simulink library "PECommon"  (Simulink 7.6)
settings: Solver=ode45  StartTime=0.0  StopTime=10.0  RelTol=1e-3
undefined symbols (not defined in the file or in its folder): DiscIntNeverNeededParam, Hydride, Metal, Nickel, Ts, Ts_Discrete
libraries: powerlib x24, simulink x14, PECommon x7, powerlib_extras x7, electricdrivelib x1, simulink_extras x1
(part 2 of 2)

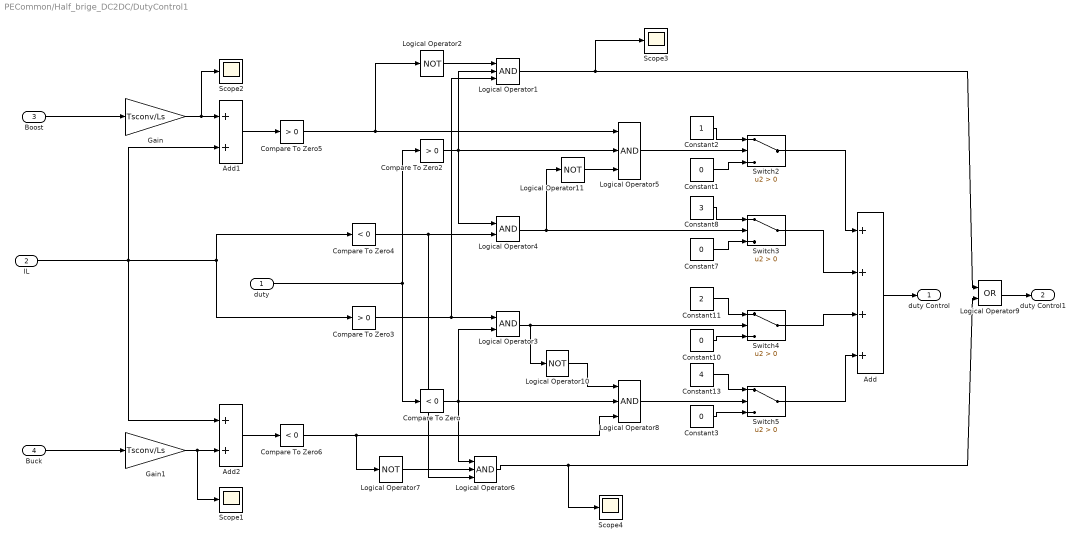
== system PECommon/Half_brige_DC2DC/DutyControl1 ==
  duty : Inport
  IL : Inport  Port=2
  Boost : Inport  Port=3
  Buck : Inport  Port=4
  Add : Sum  Inputs=++++
  Add1 : Sum
  Add2 : Sum
  Compare To Zero : simulink/Logic and Bit Operations/Compare To Zero  SystemSampleTime=-1  relop=<  LogicOutDataTypeMode=boolean  ZeroCross=off
  Compare To Zero2 : simulink/Logic and Bit Operations/Compare To Zero  SystemSampleTime=-1  relop=>  LogicOutDataTypeMode=boolean  ZeroCross=off
  Compare To Zero3 : simulink/Logic and Bit Operations/Compare To Zero  SystemSampleTime=-1  relop=>  LogicOutDataTypeMode=boolean  ZeroCross=off
  Compare To Zero4 : simulink/Logic and Bit Operations/Compare To Zero  SystemSampleTime=-1  relop=<  LogicOutDataTypeMode=boolean  ZeroCross=off
  Compare To Zero5 : simulink/Logic and Bit Operations/Compare To Zero  SystemSampleTime=-1  relop=>  LogicOutDataTypeMode=boolean  ZeroCross=off
  Compare To Zero6 : simulink/Logic and Bit Operations/Compare To Zero  SystemSampleTime=-1  relop=<  LogicOutDataTypeMode=boolean  ZeroCross=off
  Constant{1,3,7,10} (4 alike) : Constant  Value=0
  Constant11 : Constant  Value=2
  Constant13 : Constant  Value=4
  Constant2 : Constant
  Constant8 : Constant  Value=3
  Gain : Gain  Gain=Tsconv/Ls
  Gain1 : Gain  Gain=Tsconv/Ls
  Logical Operator{1,5..6,8} (4 alike) : Logic  Inputs=3  AllPortsSameDT=off  OutDataTypeStr=boolean
  Logical Operator{2,7,10..11} (4 alike) : Logic  Operator=NOT  AllPortsSameDT=off  OutDataTypeStr=boolean
  Logical Operator3 : Logic  AllPortsSameDT=off  OutDataTypeStr=boolean
  Logical Operator4 : Logic  AllPortsSameDT=off  OutDataTypeStr=boolean
  Logical Operator9 : Logic  Operator=OR  AllPortsSameDT=off  OutDataTypeStr=boolean
  Scope{1..4} (4 alike) : Scope
      Scope1 settings: SaveName=ScopeData15
      Scope2 settings: SaveName=ScopeData16
      Scope3 settings: SaveName=ScopeData17
      Scope4 settings: SaveName=ScopeData18
  Switch{2..5} (4 alike) : Switch  Criteria=u2 > Threshold  ZeroCross=off
  duty Control : Outport
  duty Control1 : Outport  Port=2
  wires:
  Constant7/1 -> Switch3/3
  Constant10/1 -> Switch4/3
  Constant11/1 -> Switch4/1
  Constant8/1 -> Switch3/1
  duty/1 -> Compare To Zero/1, Compare To Zero2/1
  Add/1 -> duty Control/1
  Constant1/1 -> Switch2/3
  Constant2/1 -> Switch2/1
  Constant3/1 -> Switch5/3
  Constant13/1 -> Switch5/1
  Compare To Zero/1 -> Logical Operator3/2, Logical Operator8/2, Logical Operator6/1
  Boost/1 -> Gain/1
  Gain/1 -> Add1/1, Scope2/1
  IL/1 -> Add1/2, Add2/1, Compare To Zero4/1, Compare To Zero3/1
  Logical Operator3/1 -> Logical Operator10/1, Switch4/2
  Compare To Zero3/1 -> Logical Operator1/3, Logical Operator3/1
  Compare To Zero2/1 -> Logical Operator4/1, Logical Operator5/2, Logical Operator1/2
  Logical Operator4/1 -> Switch3/2, Logical Operator11/1
  Compare To Zero4/1 -> Logical Operator6/3, Logical Operator4/2
  Add1/1 -> Compare To Zero5/1
  Logical Operator5/1 -> Switch2/2
  Switch3/1 -> Add/2
  Switch2/1 -> Add/1
  Buck/1 -> Gain1/1
  Add2/1 -> Compare To Zero6/1
  Gain1/1 -> Add2/2, Scope1/1
  Logical Operator8/1 -> Switch5/2
  Logical Operator10/1 -> Logical Operator8/1
  Logical Operator11/1 -> Logical Operator5/3
  Switch4/1 -> Add/3
  Switch5/1 -> Add/4
  Compare To Zero6/1 -> Logical Operator8/3, Logical Operator7/1
  Compare To Zero5/1 -> Logical Operator5/1, Logical Operator2/1
  Logical Operator2/1 -> Logical Operator1/1
  Logical Operator1/1 -> Scope3/1, Logical Operator9/1
  Logical Operator7/1 -> Logical Operator6/2
  Logical Operator6/1 -> Scope4/1, Logical Operator9/2
  Logical Operator9/1 -> duty Control1/1

== system PECommon/VSI2CSI/Value ==
  In1 : Inport
  Constant : Constant  Value=0
  Constant1 : Constant  Value=Value
  Switch : Switch  Criteria=u2 > Threshold
  Out1 : Outport
  wires:
  Switch/1 -> Out1/1
  In1/1 -> Switch/2
  Constant/1 -> Switch/3
  Constant1/1 -> Switch/1

== system PECommon/VSI2CSI/Value1 ==
  In1 : Inport
  Constant : Constant  Value=0
  Constant1 : Constant  Value=Value
  Switch : Switch  Criteria=u2 > Threshold
  Out1 : Outport
  wires:
  Constant1/1 -> Switch/1
  Constant/1 -> Switch/3
  In1/1 -> Switch/2
  Switch/1 -> Out1/1

== system PECommon/VSI2CSI/Value2 ==
  In1 : Inport
  Constant : Constant  Value=0
  Constant1 : Constant  Value=Value
  Switch : Switch  Criteria=u2 > Threshold
  Out1 : Outport
  wires:
  Switch/1 -> Out1/1
  In1/1 -> Switch/2
  Constant/1 -> Switch/3
  Constant1/1 -> Switch/1

== system PECommon/VSI2CSI/Value3 ==
  In1 : Inport
  Constant : Constant  Value=0
  Constant1 : Constant  Value=Value
  Switch : Switch  Criteria=u2 > Threshold
  Out1 : Outport
  wires:
  Constant1/1 -> Switch/1
  Constant/1 -> Switch/3
  In1/1 -> Switch/2
  Switch/1 -> Out1/1

== system PECommon/VSI2CSI/Value4 ==
  In1 : Inport
  Constant : Constant  Value=0
  Constant1 : Constant  Value=Value
  Switch : Switch  Criteria=u2 > Threshold
  Out1 : Outport
  wires:
  Switch/1 -> Out1/1
  In1/1 -> Switch/2
  Constant/1 -> Switch/3
  Constant1/1 -> Switch/1

== system PECommon/VSI2CSI/Value5 ==
  In1 : Inport
  Constant : Constant  Value=0
  Constant1 : Constant  Value=Value
  Switch : Switch  Criteria=u2 > Threshold
  Out1 : Outport
  wires:
  Constant1/1 -> Switch/1
  Constant/1 -> Switch/3
  In1/1 -> Switch/2
  Switch/1 -> Out1/1

== system PECommon/VSI2CSI/Value6 ==
  In1 : Inport
  Constant : Constant  Value=0
  Constant1 : Constant  Value=Value
  Switch : Switch  Criteria=u2 > Threshold
  Out1 : Outport
  wires:
  Constant1/1 -> Switch/1
  Constant/1 -> Switch/3
  In1/1 -> Switch/2
  Switch/1 -> Out1/1

== system PECommon/VSI2CSI/Value7 ==
  In1 : Inport
  Constant : Constant  Value=0
  Constant1 : Constant  Value=Value
  Switch : Switch  Criteria=u2 > Threshold
  Out1 : Outport
  wires:
  Switch/1 -> Out1/1
  In1/1 -> Switch/2
  Constant/1 -> Switch/3
  Constant1/1 -> Switch/1

== system PECommon/VSI2CSI/Value8 ==
  In1 : Inport
  Constant : Constant  Value=0
  Constant1 : Constant  Value=Value
  Switch : Switch  Criteria=u2 > Threshold
  Out1 : Outport
  wires:
  Constant1/1 -> Switch/1
  Constant/1 -> Switch/3
  In1/1 -> Switch/2
  Switch/1 -> Out1/1
